simulink model "PMSLM_Close_Loop_MBDL4"  (R2026a)
settings: Solver=FixedStepDiscrete  StopTime=Inf  FixedStep=Ts  EnableMultiTasking=on
values from neighbouring files (symbols this model uses):
  ADC_GainA = 0.01664    [PMSLM_Init_Params_MBDL4.m]
  ADC_GainB = 0.01664    [PMSLM_Init_Params_MBDL4.m]
  ADC_GainC = 0.01664    [PMSLM_Init_Params_MBDL4.m]
  Close_Loop_EN = Simulink.Parameter    [PMSLM_Init_Params_MBDL4.m]
  CPU_Clock = 200e6    (= 200000000)    [PMSLM_Init_Params_MBDL4.m]    (also in init_PMLSM_ThreeLoop_Simple.m)
  delay_N = 50    [PMSLM_Init_Params_MBDL4.m]
  ENCON_Manual = Simulink.Parameter    [PMSLM_Init_Params_MBDL4.m]
  FReset_Manual = Simulink.Parameter    [PMSLM_Init_Params_MBDL4.m]
  GPIO30_PWM_OE_Disable = Simulink.Parameter    [PMSLM_Init_Params_MBDL4.m]
  Grating_Resolution_mm_per_count = 0.0001    [PMSLM_Init_Params_MBDL4.m]
  Hold_Ticks = 30000    [PMSLM_Init_Params_MBDL4.m]
  Id_Init_Step = Id_Init_Target / Ramp_Ticks    (= 5e-05)    [PMSLM_Init_Params_MBDL4.m]
  Id_Init_Target = 0.5    [PMSLM_Init_Params_MBDL4.m]
  Id_Ref_Set = Simulink.Parameter    [PMSLM_Init_Params_MBDL4.m]
  Init_Reset = Simulink.Parameter    [PMSLM_Init_Params_MBDL4.m]
  Init_Start = Simulink.Parameter    [PMSLM_Init_Params_MBDL4.m]
  Iq_fric_run = 0.05    [PMSLM_Init_Params_MBDL4.m]
  Iq_fric_start = 0.40    (= 0.4)    [PMSLM_Init_Params_MBDL4.m]
  Iq_int_limit = 0.10    (= 0.1)    [PMSLM_Init_Params_MBDL4.m]    (also in init_PMLSM_ThreeLoop_Simple.m = 0.5)
  Iq_Test_Mode = Simulink.Parameter    [PMSLM_Init_Params_MBDL4.m]
  Iq_Test_Ref = Simulink.Parameter    [PMSLM_Init_Params_MBDL4.m]
  Kaw_d = Kaw_q    (= 0.2)    [PMSLM_Init_Params_MBDL4.m]    (also in init_PMLSM_ThreeLoop_Simple.m = Tuning_Gains.Kaw_d)
  Kaw_q = 0.2    [PMSLM_Init_Params_MBDL4.m]    (also in init_PMLSM_ThreeLoop_Simple.m = Tuning_Gains.Kaw_q)
  Kaw_s = 0.4    [PMSLM_Init_Params_MBDL4.m]    (also in init_PMLSM_ThreeLoop_Simple.m = Tuning_Gains.Kaw_s)
  Ki_ACR = ACR_Commissioning_Scale*Ki_ACR_Baseline    (= 2962.5)    [PMSLM_Init_Params_MBDL4.m]    (also in init_PMLSM_ThreeLoop_Simple.m = Tuning_Gains.Ki_ACR; init_PMLSM_mil_test_params.m = Kp_ACR*PMLSM_Rs_ohm/PMLSM_Lq_H)
  Ki_ASR = 0.05    [PMSLM_Init_Params_MBDL4.m]    (also in init_PMLSM_ThreeLoop_Simple.m = Tuning_Gains.Ki_ASR)
  Kp_ACR = ACR_Commissioning_Scale*Kp_ACR_Baseline    (= 2.18125)    [PMSLM_Init_Params_MBDL4.m]    (also in init_PMLSM_ThreeLoop_Simple.m = Tuning_Gains.Kp_ACR; init_PMLSM_mil_test_params.m = PMLSM_Lq_H/(4*MIL_AUM3S4_Current_PI_xi^2*MIL_AUM3S4_Current_)
  Kp_ASR = 0.03    [PMSLM_Init_Params_MBDL4.m]    (also in init_PMLSM_ThreeLoop_Simple.m = Tuning_Gains.Kp_ASR)
  Kp_pos = 5    [PMSLM_Init_Params_MBDL4.m]    (also in init_PMLSM_ThreeLoop_Simple.m = Tuning_Gains.Kp_pos)
  OffsetCal_EN = Simulink.Parameter    [PMSLM_Init_Params_MBDL4.m]
  PI_Reset_EN = Simulink.Parameter    [PMSLM_Init_Params_MBDL4.m]
  PMLSM_Ld_H = Ld    (= 0.001745)    [PMSLM_Init_Params_MBDL4.m]    (also in init_PMLSM_ThreeLoop_Simple.m; init_PMLSM_plant_params.m)
  PMLSM_Lq_H = Lq    (= 0.001745)    [PMSLM_Init_Params_MBDL4.m]    (also in init_PMLSM_ThreeLoop_Simple.m; init_PMLSM_plant_params.m)
  PMLSM_psi_f_Wb = flux    (= 0.141)    [PMSLM_Init_Params_MBDL4.m]    (also in init_PMLSM_ThreeLoop_Simple.m; init_PMLSM_plant_params.m)
  Pos_deadband = 0.02    [PMSLM_Init_Params_MBDL4.m]    (also in init_PMLSM_ThreeLoop_Simple.m)
  Pos_Loop_EN = Simulink.Parameter    [PMSLM_Init_Params_MBDL4.m]
  qep_mid_cnt = 2147483648    [PMSLM_Init_Params_MBDL4.m]
  Ramp_Ticks = 10000    [PMSLM_Init_Params_MBDL4.m]
  RELCON_Manual = Simulink.Parameter    [PMSLM_Init_Params_MBDL4.m]
  Speed_loop_Iq_Limit = Iq_Limit    (= 0.3)    [PMSLM_Init_Params_MBDL4.m]    (also in init_PMLSM_ThreeLoop_Simple.m = 1)
  Tau_e_mm = 60    [PMSLM_Init_Params_MBDL4.m]
  theta_align_const = 0    [PMSLM_Init_Params_MBDL4.m]
  Theta_Offset_Fine = Simulink.Parameter    [PMSLM_Init_Params_MBDL4.m]
  Three_Current_Sampling_EN = Simulink.Parameter    [PMSLM_Init_Params_MBDL4.m]
  Ts = 1 / PWM_Freq    (= 0.0001)    [PMSLM_Init_Params_MBDL4.m]    (also in init_PMLSM_ThreeLoop_Simple.m)
  Ts_ACR = 1e-4    (= 0.0001)    [PMSLM_Init_Params_MBDL4.m]    (also in init_PMLSM_ThreeLoop_Simple.m)
  Ts_ASR = 1e-3    (= 0.001)    [PMSLM_Init_Params_MBDL4.m]    (also in init_PMLSM_ThreeLoop_Simple.m)
  Udc = 48    [PMSLM_Init_Params_MBDL4.m]    (also in init_PMLSM_ThreeLoop_Simple.m; init_PMLSM_mil_test_params.m)
  Uq_Zero_EN = 0：q 轴用正常 PI    [PMSLM_Init_Params_MBDL4.m]
  v_ff_eps = 0.5    [PMSLM_Init_Params_MBDL4.m]    (also in init_PMLSM_ThreeLoop_Simple.m)
  V_meas_max = 500    [PMSLM_Init_Params_MBDL4.m]
  v_meas_zero_eps = 0.5    [PMSLM_Init_Params_MBDL4.m]
  v_over_eps = 3    [PMSLM_Init_Params_MBDL4.m]    (also in init_PMLSM_ThreeLoop_Simple.m)
  V_pos_max_mmps = 10    [PMSLM_Init_Params_MBDL4.m]    (also in init_PMLSM_ThreeLoop_Simple.m = 20)
  v_ref_max = 20    [PMSLM_Init_Params_MBDL4.m]    (also in init_PMLSM_ThreeLoop_Simple.m)
  v_ref_set = Simulink.Parameter    [PMSLM_Init_Params_MBDL4.m]
  v_ref_set_step_dn = v_ref_set_rate_dn * Ts    (= 0.005)    [PMSLM_Init_Params_MBDL4.m]    (also in init_PMLSM_ThreeLoop_Simple.m)
  v_ref_set_step_up = v_ref_set_rate_up * Ts    (= 0.005)    [PMSLM_Init_Params_MBDL4.m]    (also in init_PMLSM_ThreeLoop_Simple.m)
  v_ref_zero_eps = 0.2    [PMSLM_Init_Params_MBDL4.m]    (also in init_PMLSM_ThreeLoop_Simple.m = 0)
  v_stick_off = 3.0    (= 3)    [PMSLM_Init_Params_MBDL4.m]
  v_stick_on = 1.0    (= 1)    [PMSLM_Init_Params_MBDL4.m]
  X_max_hard = 500    [PMSLM_Init_Params_MBDL4.m]
  X_max_soft = 470    [PMSLM_Init_Params_MBDL4.m]
  X_min_hard = -500    [PMSLM_Init_Params_MBDL4.m]
  X_min_soft = -470    [PMSLM_Init_Params_MBDL4.m]
  x_ref_mm = Simulink.Parameter    [PMSLM_Init_Params_MBDL4.m]
undefined symbols (not defined in the file or in its folder): bit, Down, GPTRIP1SEL, TZ1, Up
libraries: simulink x11, c2802xlib x6, c2838xlib x6, mcbeeMathTransformLib x2, c280xlib x1, mcbcontrolslib x1, svdschedulerlib x1
(part 2 of 2)

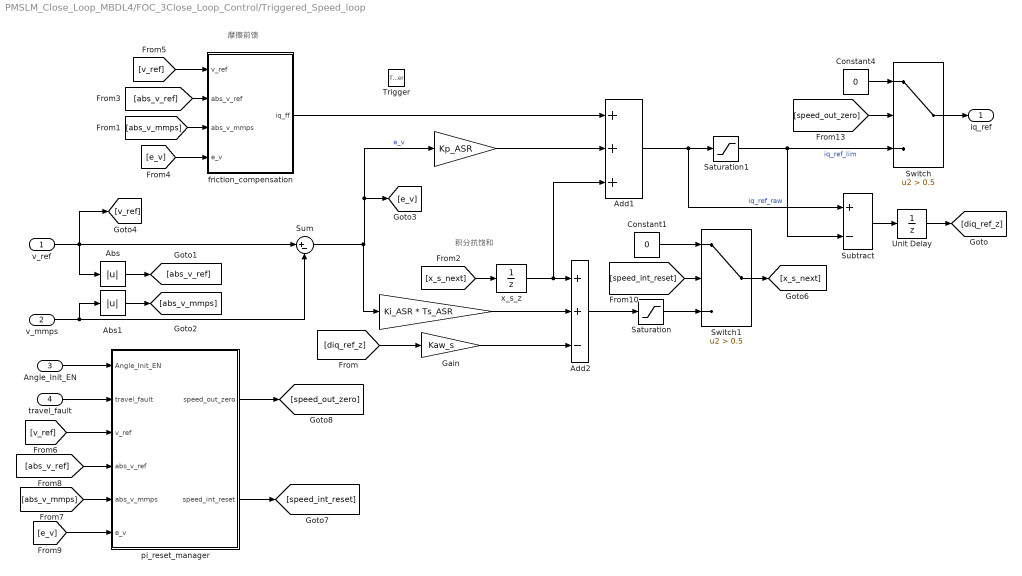
== system PMSLM_Close_Loop_MBDL4/FOC_3Close_Loop_Control/Triggered_Speed_loop ==
  note: 摩擦前馈
  note: 积分抗饱和
  v_ref : Inport
  v_mmps : Inport  Port=2
  Angle_Init_EN : Inport  Port=3
  travel_fault : Inport  Port=4
  Trigger : TriggerPort  VariantControl=(inherit)
  " " : Gain  Gain=Ki_ASR * Ts_ASR
  "  " : Gain  Gain=Kp_ASR
  Abs : Abs  SaturateOnIntegerOverflow=off
  Abs1 : Abs  SaturateOnIntegerOverflow=off
  Add1 : Sum  Inputs=+++
  Add2 : Sum  Inputs=++-
  Constant1 : Constant  Value=0
  Constant4 : Constant  Value=0
  Gain : Gain  Gain=Kaw_s
  Saturation : Saturate  UpperLimit=Iq_int_limit  LowerLimit=-Iq_int_limit
  Saturation1 : Saturate  UpperLimit=Speed_loop_Iq_Limit  LowerLimit=-Speed_loop_Iq_Limit
  Subtract : Sum  Inputs=+-
  Sum : Sum  Inputs=|+-
  Switch : Switch  Criteria=u2 > Threshold  Threshold=0.5  SaturateOnIntegerOverflow=off  InputSameDT=off
  Switch1 : Switch  Criteria=u2 > Threshold  Threshold=0.5  SaturateOnIntegerOverflow=off  InputSameDT=off
  Unit Delay : UnitDelay  SampleTime=-1
  friction_compensation : Subsystem
  pi_reset_manager : Subsystem
  x_s_z : UnitDelay  SampleTime=-1
  iq_ref : Outport
  wires:
  v_mmps/1 -> Sum/2, Abs1/1
  Sum/1 -> " "/1, [e_v], "  "/1  "e_v"
  Add1/1 -> Subtract/1, Saturation1/1  "iq_ref_raw"
  v_ref/1 -> [v_ref], Abs/1, Sum/1
  Saturation1/1 -> Subtract/2, Switch/3  "iq_ref_lim"
  [x_s_next] -> x_s_z/1
  Add2/1 -> Saturation/1
  Gain/1 -> Add2/3
  " "/1 -> Add2/2
  Subtract/1 -> Unit Delay/1
  Unit Delay/1 -> [diq_ref_z]
  [diq_ref_z] -> Gain/1
  Constant1/1 -> Switch1/1
  Switch/1 -> iq_ref/1
  Constant4/1 -> Switch/1
  "  "/1 -> Add1/2
  friction_compensation/1(iq_ff) -> Add1/1
  x_s_z/1 -> Add1/3, Add2/1
  [e_v] -> friction_compensation/4(e_v)
  [abs_v_mmps] -> friction_compensation/3(abs_v_mmps)
  [abs_v_ref] -> friction_compensation/2(abs_v_ref)
  Abs/1 -> [abs_v_ref]
  Abs1/1 -> [abs_v_mmps]
  Angle_Init_EN/1 -> pi_reset_manager/1(Angle_Init_EN)
  travel_fault/1 -> pi_reset_manager/2(travel_fault)
  [v_ref] -> friction_compensation/1(v_ref)
  [v_ref] -> pi_reset_manager/3(v_ref)
  [abs_v_mmps] -> pi_reset_manager/5(abs_v_mmps)
  [abs_v_ref] -> pi_reset_manager/4(abs_v_ref)
  [e_v] -> pi_reset_manager/6(e_v)
  [speed_out_zero] -> Switch/2
  pi_reset_manager/2(speed_int_reset) -> [speed_int_reset]
  pi_reset_manager/1(speed_out_zero) -> [speed_out_zero]
  [speed_int_reset] -> Switch1/2
  Switch1/1 -> [x_s_next]
  Saturation/1 -> Switch1/3

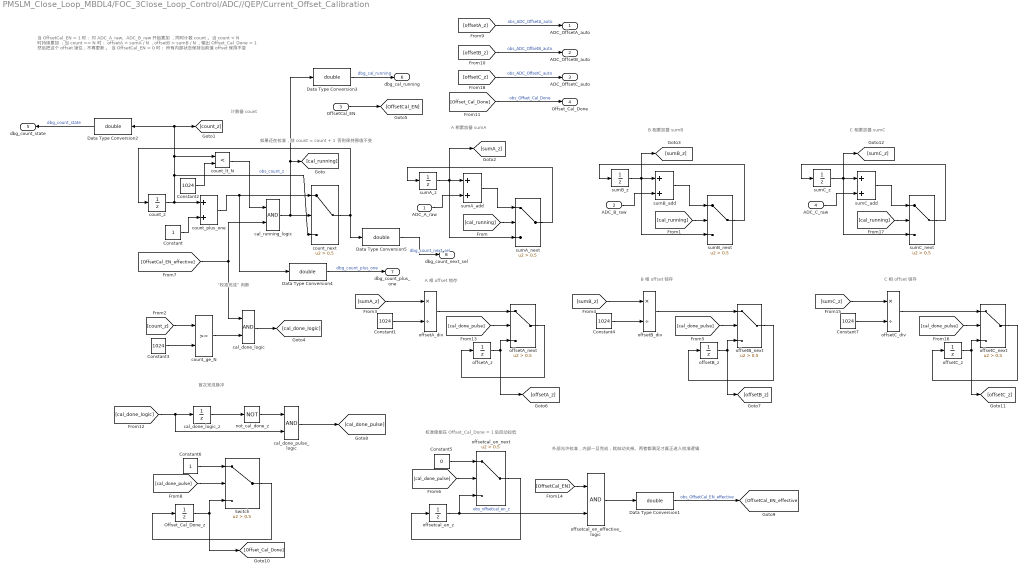
== system PMSLM_Close_Loop_MBDL4/FOC_3Close_Loop_Control/ADC//QEP/Current_Offset_Calibration ==
  note: 校准使能在 Offset_Cal_Done = 1 后自动拉低
  note: 外部允许校准，内部一旦完成，就自动关掉。两者都满足才真正进入校准逻辑
  note: 首次完成脉冲
  note: “校准完成” 判断
  note: B 相累加器 sumB
  note: A 相累加器 sumA
  note: 计数器 count
  note: B 相 offset 锁存
  note: A 相 offset 锁存
  note: 如果还在校准，就 count = count + 1 否则保持原值不变
  note: 当 OffsetCal_EN = 1 时：
      | 对 ADC_A_raw、ADC_B_raw 开始累加 ，同时计数 count 。当 count < N 时持续累加 ；当 count == N 时： offsetA = sumA / N ，offsetB = sumB / N ，输出 Offset_Cal_Done = 1 然后把这个 offset 锁住，不再更新 。
      |
      | 当 OffsetCal_EN = 0 时：
      | 所有内部状态保持当前值 offset 保持不变
  note: C 相 offset 锁存
  note: C 相累加器 sumC
  ADC_A_raw : Inport
  ADC_B_raw : Inport  Port=2
  OffsetCal_EN : Inport  Port=3
  ADC_C_raw : Inport  Port=4
  Constant : Constant  OutDataTypeStr=double
  Constant{1..4,7} (5 alike) : Constant  Value=1024  OutDataTypeStr=double
  Constant5 : Constant  Value=0  OutDataTypeStr=double
  Constant6 : Constant  OutDataTypeStr=double
  Data Type Conversion{1..5} (5 alike) : DataTypeConversion  OutDataTypeStr=double  SaturateOnIntegerOverflow=off  RndMeth=Floor
  Offset_Cal_Done_z : UnitDelay  SampleTime=-1
  Switch : Switch  Criteria=u2 > Threshold  Threshold=0.5  OutDataTypeStr=double  SaturateOnIntegerOverflow=off  InputSameDT=off
  cal_done_logic : Logic  AllPortsSameDT=off  OutDataTypeStr=boolean
  cal_done_logic_z : UnitDelay  SampleTime=-1
  cal_done_pulse_logic : Logic  AllPortsSameDT=off  OutDataTypeStr=boolean
  cal_running_logic : Logic  AllPortsSameDT=off  OutDataTypeStr=boolean
  count_ge_N : RelationalOperator  OutDataTypeStr=boolean  RndMeth=Simplest  InputSameDT=off
  count_lt_N : RelationalOperator  Operator=<  OutDataTypeStr=boolean  RndMeth=Simplest  InputSameDT=off
  count_next : Switch  Criteria=u2 > Threshold  Threshold=0.5  OutDataTypeStr=double  SaturateOnIntegerOverflow=off  InputSameDT=off
  count_plus_one : Sum
  count_z : UnitDelay  SampleTime=-1
  not_cal_done_z : Logic  Operator=NOT  AllPortsSameDT=off  OutDataTypeStr=boolean
  offsetA_div : Product  Inputs=*/
  offsetA_next : Switch  Criteria=u2 > Threshold  Threshold=0.5  OutDataTypeStr=double  SaturateOnIntegerOverflow=off  InputSameDT=off
  offsetA_z : UnitDelay  InitialCondition=2253  SampleTime=-1
  offsetB_div : Product  Inputs=*/
  offsetB_next : Switch  Criteria=u2 > Threshold  Threshold=0.5  OutDataTypeStr=double  SaturateOnIntegerOverflow=off  InputSameDT=off
  offsetB_z : UnitDelay  InitialCondition=2253  SampleTime=-1
  offsetC_div : Product  Inputs=*/
  offsetC_next : Switch  Criteria=u2 > Threshold  Threshold=0.5  OutDataTypeStr=double  SaturateOnIntegerOverflow=off  InputSameDT=off
  offsetC_z : UnitDelay  InitialCondition=2253  SampleTime=-1
  offsetcal_en_effective_logic : Logic  AllPortsSameDT=off  OutDataTypeStr=boolean
  offsetcal_en_next : Switch  Criteria=u2 > Threshold  Threshold=0.5  OutDataTypeStr=double  SaturateOnIntegerOverflow=off  InputSameDT=off
  offsetcal_en_z : UnitDelay  InitialCondition=1  SampleTime=-1
  sumA_add : Sum
  sumA_next : Switch  Criteria=u2 > Threshold  Threshold=0.5  OutDataTypeStr=double  SaturateOnIntegerOverflow=off  InputSameDT=off
  sumA_z : UnitDelay  SampleTime=-1
  sumB_add : Sum
  sumB_next : Switch  Criteria=u2 > Threshold  Threshold=0.5  OutDataTypeStr=double  SaturateOnIntegerOverflow=off  InputSameDT=off
  sumB_z : UnitDelay  SampleTime=-1
  sumC_add : Sum
  sumC_next : Switch  Criteria=u2 > Threshold  Threshold=0.5  OutDataTypeStr=double  SaturateOnIntegerOverflow=off  InputSameDT=off
  sumC_z : UnitDelay  SampleTime=-1
  ADC_OffsetA_auto : Outport
  ADC_OffsetB_auto : Outport  Port=2
  ADC_OffsetC_auto : Outport  Port=3
  Offset_Cal_Done : Outport  Port=4
  dbg_count_state : Outport  Port=5
  dbg_cal_running : Outport  Port=6
  dbg_count_plus_one : Outport  Port=7
  dbg_count_next_sel : Outport  Port=8
  wires:
  count_z/1 -> Data Type Conversion2/1, [count_z], count_lt_N/1, count_next/3, count_plus_one/1  "obs_count_z"
  Constant/1 -> count_plus_one/2
  Constant2/1 -> count_lt_N/2
  count_lt_N/1 -> cal_running_logic/1
  count_plus_one/1 -> Data Type Conversion4/1, count_next/1
  cal_running_logic/1 -> Data Type Conversion3/1, [cal_running], count_next/2
  count_next/1 -> count_z/1, Data Type Conversion5/1
  sumA_z/1 -> [sumA_z], sumA_next/3, sumA_add/1
  ADC_A_raw/1 -> sumA_add/2
  sumA_add/1 -> sumA_next/1
  [cal_running] -> sumA_next/2
  sumA_next/1 -> sumA_z/1
  sumB_next/1 -> sumB_z/1
  [cal_running] -> sumB_next/2
  sumB_add/1 -> sumB_next/1
  ADC_B_raw/1 -> sumB_add/2
  sumB_z/1 -> [sumB_z], sumB_next/3, sumB_add/1
  [count_z] -> count_ge_N/1
  Constant3/1 -> count_ge_N/2
  count_ge_N/1 -> cal_done_logic/2
  [sumA_z] -> offsetA_div/1
  Constant1/1 -> offsetA_div/2
  Constant4/1 -> offsetB_div/2
  [sumB_z] -> offsetB_div/1
  offsetA_div/1 -> offsetA_next/1
  cal_done_logic/1 -> [cal_done_logic]
  offsetA_z/1 -> [offsetA_z], offsetA_next/3
  offsetA_next/1 -> offsetA_z/1
  [cal_done_pulse] -> offsetB_next/2
  offsetB_z/1 -> [offsetB_z], offsetB_next/3
  offsetB_next/1 -> offsetB_z/1
  offsetB_div/1 -> offsetB_next/1
  OffsetCal_EN/1 -> [OffsetCal_EN]
  [offsetA_z] -> ADC_OffsetA_auto/1  "obs_ADC_OffsetA_auto"
  [offsetB_z] -> ADC_OffsetB_auto/1  "obs_ADC_OffsetB_auto"
  [cal_done_logic] -> cal_done_pulse_logic/2, cal_done_logic_z/1
  cal_done_logic_z/1 -> not_cal_done_z/1
  not_cal_done_z/1 -> cal_done_pulse_logic/1
  [cal_done_pulse] -> offsetA_next/2
  Constant5/1 -> offsetcal_en_next/1
  [cal_done_pulse] -> offsetcal_en_next/2
  offsetcal_en_z/1 -> offsetcal_en_effective_logic/2, offsetcal_en_next/3  "obs_offsetcal_en_z"
  offsetcal_en_next/1 -> offsetcal_en_z/1
  [OffsetCal_EN] -> offsetcal_en_effective_logic/1
  offsetcal_en_effective_logic/1 -> Data Type Conversion1/1
  [OffsetCal_EN_effective] -> cal_running_logic/2, cal_done_logic/1
  [Offset_Cal_Done] -> Offset_Cal_Done/1  "obs_Offset_Cal_Done"
  Data Type Conversion1/1 -> [OffsetCal_EN_effective]  "obs_OffsetCal_EN_effective"
  Data Type Conversion2/1 -> dbg_count_state/1  "dbg_count_state"
  Data Type Conversion3/1 -> dbg_cal_running/1  "dbg_cal_running"
  Data Type Conversion4/1 -> dbg_count_plus_one/1  "dbg_count_plus_one"
  Data Type Conversion5/1 -> dbg_count_next_sel/1  "dbg_count_next_sel"
  cal_done_pulse_logic/1 -> [cal_done_pulse]
  Constant6/1 -> Switch/1
  [cal_done_pulse] -> Switch/2
  Offset_Cal_Done_z/1 -> [Offset_Cal_Done], Switch/3
  Switch/1 -> Offset_Cal_Done_z/1
  offsetC_z/1 -> [offsetC_z], offsetC_next/3
  Constant7/1 -> offsetC_div/2
  [sumC_z] -> offsetC_div/1
  offsetC_div/1 -> offsetC_next/1
  offsetC_next/1 -> offsetC_z/1
  [cal_done_pulse] -> offsetC_next/2
  sumC_z/1 -> [sumC_z], sumC_next/3, sumC_add/1
  ADC_C_raw/1 -> sumC_add/2
  sumC_add/1 -> sumC_next/1
  sumC_next/1 -> sumC_z/1
  [cal_running] -> sumC_next/2
  [offsetC_z] -> ADC_OffsetC_auto/1  "obs_ADC_OffsetC_auto"

== system PMSLM_Close_Loop_MBDL4/FOC_3Close_Loop_Control/Caculate_measurement/IIR Filter ==
  In1 : Inport
  Reset : ResetPort  DisableCoverage=on
  IIR Filter : mcbcontrolslib/IIR Filter  VariantControl=Low Pass Filter  VariantSelect=Low-pass  FilterConstantInputType=Specify via dialog  Filter_constant=0.1  InitialOutput=Specify via dialog  InitialOutputValue=0  ExternalReset=none  advancedSettings=on  Ts=100e-6  cutOff_freq=176.8388
  Out1 : Outport
  wires:
  In1/1 -> IIR Filter/1
  IIR Filter/1 -> Out1/1

== system PMSLM_Close_Loop_MBDL4/FOC_3Close_Loop_Control/Controller_Driver_IO_Manager/External_Fault_Latch ==
  ERRI_raw : Inport  OutDataTypeStr=boolean  PortDimensions=1
  ERRU_raw : Inport  Port=2  OutDataTypeStr=boolean  PortDimensions=1
  ERRI_Active_Low : Logic  Operator=NOT  IconShape=distinctive
  ERRU_Active_Low : Logic  Operator=NOT  IconShape=distinctive
  External_Fault_Latch_OR : Logic  Operator=OR  IconShape=distinctive
  External_Fault_Latch_Z : UnitDelay  InitialCondition=false  SampleTime=-1
  External_Fault_OR : Logic  Operator=OR  IconShape=distinctive
  external_fault_latch : Outport  OutDataTypeStr=boolean  PortDimensions=1
  wires:
  External_Fault_Latch_OR/1 -> External_Fault_Latch_Z/1, external_fault_latch/1
  External_Fault_Latch_Z/1 -> External_Fault_Latch_OR/2
  External_Fault_OR/1 -> External_Fault_Latch_OR/1
  ERRU_Active_Low/1 -> External_Fault_OR/2
  ERRI_Active_Low/1 -> External_Fault_OR/1
  ERRU_raw/1 -> ERRU_Active_Low/1
  ERRI_raw/1 -> ERRI_Active_Low/1

== system PMSLM_Close_Loop_MBDL4/FOC_3Close_Loop_Control/FOC_Algorithm/Clack ==
  note: alpha=(A-0.5*(B+C))*2/3
      | Beta=sqrt(3)/2*(B-C)*2/3
  ia : Inport
  ib : Inport  Port=2
  ic : Inport  Port=3
  Add : Sum  Inputs=+--
  Add1 : Sum  Inputs=+-
  Gain : Gain  Gain=0.5
  Gain1 : Gain  Gain=0.5
  Gain2 : Gain  Gain=2/3
  Gain3 : Gain  Gain=1/sqrt(3)
  ialpha : Outport
  ibeta : Outport  Port=2
  wires:
  Gain1/1 -> Add/3
  ia/1 -> Add/1
  ib/1 -> Add1/1, Gain/1
  Add1/1 -> Gain3/1
  ic/1 -> Add1/2, Gain1/1
  Gain3/1 -> ibeta/1  "ibeta"
  Add/1 -> Gain2/1
  Gain2/1 -> ialpha/1  "ialf"
  Gain/1 -> Add/2

== system PMSLM_Close_Loop_MBDL4/FOC_3Close_Loop_Control/FOC_Algorithm/SVPWMG ==
  Valpha : Inport
  Vbeta : Inport  Port=2
  Duty Calculate : Subsystem  TreatAsAtomicUnit=on  RTWFcnName=Duty_Caculate_Fun
      settings: RTWFcnNameOpts=User specified
  Sector Caculate : Subsystem  TreatAsAtomicUnit=on  RTWFcnName=Sector_Caculate_Fun
      settings: RTWFcnNameOpts=User specified
  T1T2 Calculate : Subsystem  TreatAsAtomicUnit=on  RTWFcnName=T1T2Caculate_Fun
      settings: RTWFcnNameOpts=User specified
  Udc : Constant  Value=Udc
  XYZ Calculate : Subsystem  TreatAsAtomicUnit=on  RTWFcnName=XYZ_Caculate_Fun
      settings: RTWFcnNameOpts=User specified
  Duty_A : Outport
  Duty_B : Outport  Port=2
  Duty_C : Outport  Port=3
  "N " : Outport  Port=4
  wires:
  Vbeta/1 -> Sector Caculate/2(Ubeta), XYZ Calculate/2(Ubeta)
  T1T2 Calculate/1(T1) -> Duty Calculate/2(T1)
  Valpha/1 -> Sector Caculate/1(Ualpha), XYZ Calculate/1(Ualpha)
  T1T2 Calculate/2(T2) -> Duty Calculate/3(T2)
  Sector Caculate/1("N ") -> "N "/1, Duty Calculate/1(N), T1T2 Calculate/1(N)
  Udc/1 -> XYZ Calculate/3(Udc)
  XYZ Calculate/1(X) -> T1T2 Calculate/2(X)
  XYZ Calculate/2(Y) -> T1T2 Calculate/3(Y)
  XYZ Calculate/3(Z) -> T1T2 Calculate/4(Z)
  Duty Calculate/1(Duty_U) -> Duty_A/1
  Duty Calculate/2(Duty_V) -> Duty_B/1
  Duty Calculate/3(Duty_W) -> Duty_C/1

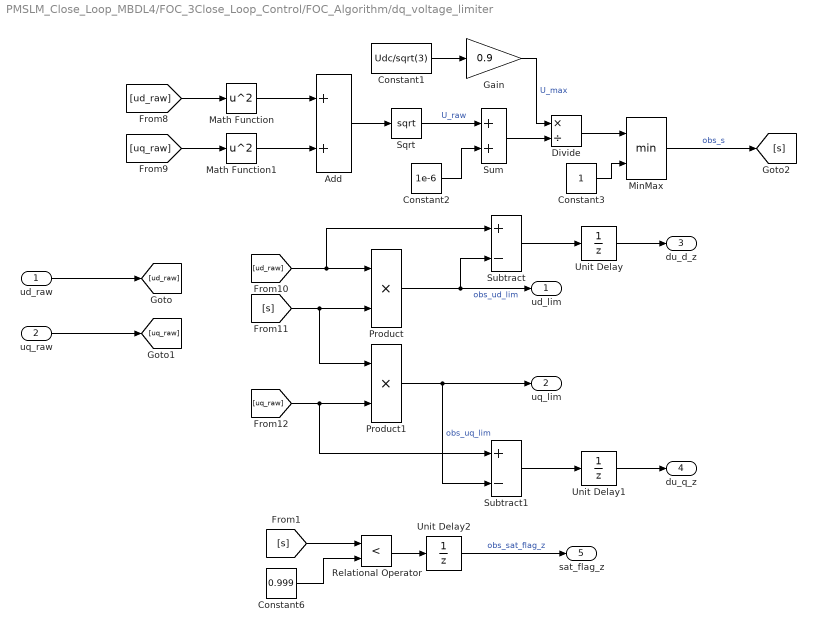
== system PMSLM_Close_Loop_MBDL4/FOC_3Close_Loop_Control/FOC_Algorithm/dq_voltage_limiter ==
  ud_raw : Inport
  uq_raw : Inport  Port=2
  Add : Sum
  Constant1 : Constant  Value=Udc/sqrt(3)  OutDataTypeStr=double
  Constant2 : Constant  Value=1e-6  OutDataTypeStr=double
  Constant3 : Constant  OutDataTypeStr=double
  Constant6 : Constant  Value=0.999
  Divide : Product  Inputs=*/  OutDataTypeStr=double
  Gain : Gain  Gain=0.9  OutDataTypeStr=double
  Math Function : Math  Operator=square
  Math Function1 : Math  Operator=square
  MinMax : MinMax  Inputs=2
  Product : Product
  Product1 : Product  OutDataTypeStr=double
  Relational Operator : RelationalOperator  Operator=<  OutDataTypeStr=boolean  RndMeth=Simplest  InputSameDT=off
  Sqrt : Sqrt
  Subtract : Sum  Inputs=+-
  Subtract1 : Sum  Inputs=+-
  Sum : Sum
  Unit Delay : UnitDelay  SampleTime=-1
  Unit Delay1 : UnitDelay  SampleTime=-1
  Unit Delay2 : UnitDelay  SampleTime=-1
  ud_lim : Outport
  uq_lim : Outport  Port=2
  du_d_z : Outport  Port=3
  du_q_z : Outport  Port=4
  sat_flag_z : Outport  Port=5
  wires:
  Sum/1 -> Divide/2
  Constant2/1 -> Sum/2
  Constant3/1 -> MinMax/2
  Add/1 -> Sqrt/1
  Constant1/1 -> Gain/1
  Divide/1 -> MinMax/1
  Gain/1 -> Divide/1  "U_max"
  Sqrt/1 -> Sum/1  "U_raw"
  Math Function1/1 -> Add/2
  Math Function/1 -> Add/1
  [uq_raw] -> Math Function1/1
  [ud_raw] -> Math Function/1
  MinMax/1 -> [s]  "obs_s"
  Product1/1 -> uq_lim/1, Subtract1/2  "obs_uq_lim"
  [s] -> Product1/1, Product/2
  [ud_raw] -> Subtract/1, Product/1
  Product/1 -> Subtract/2, ud_lim/1  "obs_ud_lim"
  [uq_raw] -> Subtract1/1, Product1/2
  Subtract/1 -> Unit Delay/1
  Subtract1/1 -> Unit Delay1/1
  ud_raw/1 -> [ud_raw]
  uq_raw/1 -> [uq_raw]
  Unit Delay/1 -> du_d_z/1
  Unit Delay1/1 -> du_q_z/1
  Constant6/1 -> Relational Operator/2
  [s] -> Relational Operator/1
  Relational Operator/1 -> Unit Delay2/1
  Unit Delay2/1 -> sat_flag_z/1  "obs_sat_flag_z"

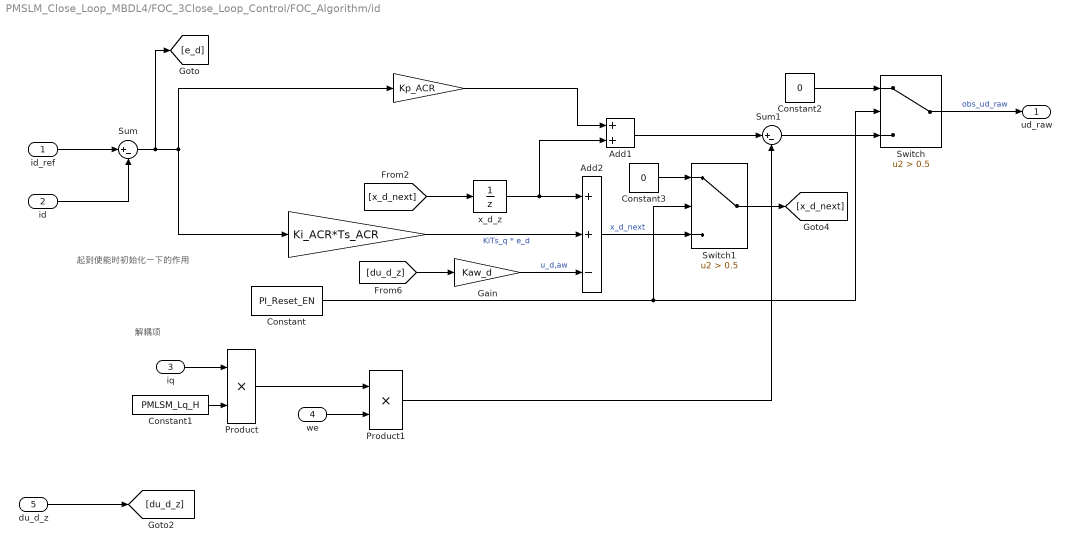
== system PMSLM_Close_Loop_MBDL4/FOC_3Close_Loop_Control/FOC_Algorithm/id ==
  note: 解耦项
  note: 起到使能时初始化一下的作用
  id_ref : Inport
  id : Inport  Port=2
  iq : Inport  Port=3
  we : Inport  Port=4
  du_d_z : Inport  Port=5
  " " : Gain  Gain=Ki_ACR*Ts_ACR
  "  " : Gain  Gain=Kp_ACR
  Add1 : Sum
  Add2 : Sum  Inputs=++-
  Constant : Constant  Value=PI_Reset_EN
  Constant1 : Constant  Value=PMLSM_Lq_H
  Constant2 : Constant  Value=0
  Constant3 : Constant  Value=0
  Gain : Gain  Gain=Kaw_d
  Product : Product
  Product1 : Product
  Sum : Sum  Inputs=|+-
  Sum1 : Sum  Inputs=|+-
  Switch : Switch  Criteria=u2 > Threshold  Threshold=0.5  SaturateOnIntegerOverflow=off  InputSameDT=off
  Switch1 : Switch  Criteria=u2 > Threshold  Threshold=0.5  SaturateOnIntegerOverflow=off  InputSameDT=off
  x_d_z : UnitDelay  SampleTime=-1
  ud_raw : Outport
  wires:
  iq/1 -> Product/1
  id_ref/1 -> Sum/1
  id/1 -> Sum/2
  Sum/1 -> [e_d], " "/1, "  "/1
  Product1/1 -> Sum1/2
  we/1 -> Product1/2
  Product/1 -> Product1/1
  Add1/1 -> Sum1/1
  Constant1/1 -> Product/2
  Constant/1 -> Switch1/2, Switch/2
  "  "/1 -> Add1/1
  Constant2/1 -> Switch/1
  Sum1/1 -> Switch/3
  Switch/1 -> ud_raw/1  "obs_ud_raw"
  du_d_z/1 -> [du_d_z]
  x_d_z/1 -> Add1/2, Add2/1
  [x_d_next] -> x_d_z/1
  Add2/1 -> Switch1/3  "x_d_next"
  Gain/1 -> Add2/3  "u_d,aw"
  [du_d_z] -> Gain/1
  " "/1 -> Add2/2  "KiTs_q * e_d"
  Constant3/1 -> Switch1/1
  Switch1/1 -> [x_d_next]

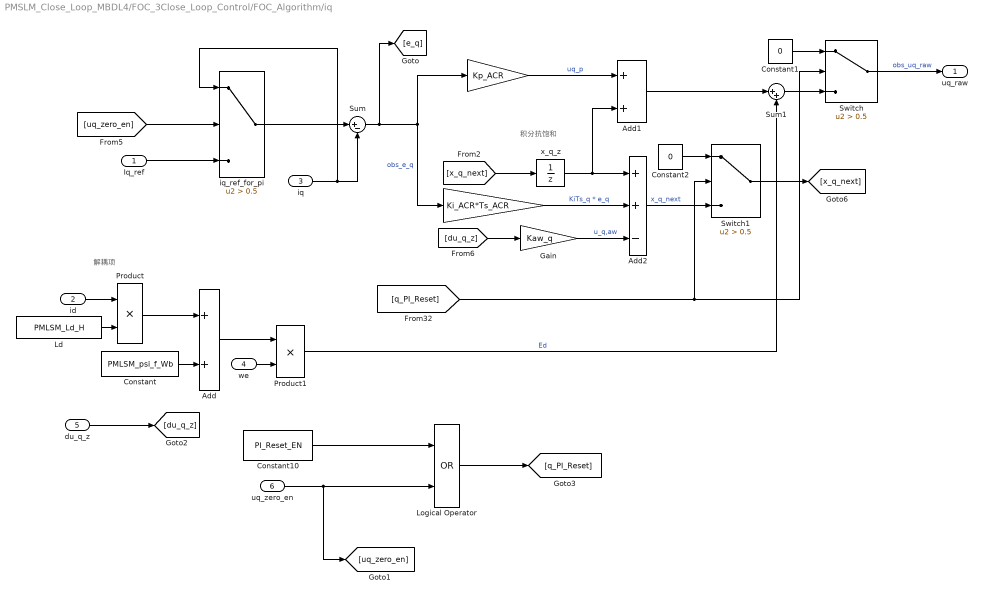
== system PMSLM_Close_Loop_MBDL4/FOC_3Close_Loop_Control/FOC_Algorithm/iq ==
  note: 解耦项
  note: 积分抗饱和
  Iq_ref : Inport
  id : Inport  Port=2
  iq : Inport  Port=3
  we : Inport  Port=4
  du_q_z : Inport  Port=5
  uq_zero_en : Inport  Port=6
  " " : Gain  Gain=Ki_ACR*Ts_ACR
  "  " : Gain  Gain=Kp_ACR
  Add : Sum
  Add1 : Sum
  Add2 : Sum  Inputs=++-
  Constant : Constant  Value=PMLSM_psi_f_Wb
  Constant1 : Constant  Value=0
  Constant10 : Constant  Value=PI_Reset_EN
  Constant2 : Constant  Value=0
  Gain : Gain  Gain=Kaw_q
  Ld : Constant  Value=PMLSM_Ld_H
  Logical Operator : Logic  Operator=OR  AllPortsSameDT=off  OutDataTypeStr=boolean
  Product : Product
  Product1 : Product
  Sum : Sum  Inputs=|+-
  Sum1 : Sum  Inputs=|++
  Switch : Switch  Criteria=u2 > Threshold  Threshold=0.5  SaturateOnIntegerOverflow=off  InputSameDT=off
  Switch1 : Switch  Criteria=u2 > Threshold  Threshold=0.5  SaturateOnIntegerOverflow=off  InputSameDT=off
  iq_ref_for_pi : Switch  Criteria=u2 > Threshold  Threshold=0.5  SaturateOnIntegerOverflow=off  InputSameDT=off
  x_q_z : UnitDelay  SampleTime=-1
  uq_raw : Outport
  wires:
  Product1/1 -> Sum1/2  "Ed"
  we/1 -> Product1/2
  Add1/1 -> Sum1/1
  iq/1 -> iq_ref_for_pi/1, Sum/2
  id/1 -> Product/1
  Ld/1 -> Product/2
  Product/1 -> Add/1
  Constant/1 -> Add/2
  Add/1 -> Product1/1
  Sum/1 -> [e_q], "  "/1, " "/1  "obs_e_q"
  "  "/1 -> Add1/1  "uq_p"
  Constant1/1 -> Switch/1
  Switch/1 -> uq_raw/1  "obs_uq_raw"
  Sum1/1 -> Switch/3
  [q_PI_Reset] -> Switch/2, Switch1/2
  du_q_z/1 -> [du_q_z]
  [uq_zero_en] -> iq_ref_for_pi/2
  Iq_ref/1 -> iq_ref_for_pi/3
  iq_ref_for_pi/1 -> Sum/1
  [du_q_z] -> Gain/1
  Gain/1 -> Add2/3  "u_q,aw"
  " "/1 -> Add2/2  "KiTs_q * e_q"
  x_q_z/1 -> Add1/2, Add2/1
  Constant2/1 -> Switch1/1
  Add2/1 -> Switch1/3  "x_q_next"
  Switch1/1 -> [x_q_next]
  [x_q_next] -> x_q_z/1
  uq_zero_en/1 -> [uq_zero_en], Logical Operator/2
  Constant10/1 -> Logical Operator/1
  Logical Operator/1 -> [q_PI_Reset]

== system PMSLM_Close_Loop_MBDL4/FOC_3Close_Loop_Control/Reference_Manager/v_ref_set_slew_limiter ==
  v_ref_set : Inport
  Add : Sum
  Saturation : Saturate  UpperLimit=v_ref_set_step_up  LowerLimit=-v_ref_set_step_dn
  Subtract : Sum  Inputs=+-
  v_ref_set_lim_z : UnitDelay  SampleTime=-1
  v_ref_set_limited : Outport
  wires:
  v_ref_set_lim_z/1 -> Add/2, Subtract/2
  v_ref_set/1 -> Subtract/1
  Saturation/1 -> Add/1
  Subtract/1 -> Saturation/1
  Add/1 -> v_ref_set_limited/1, v_ref_set_lim_z/1

== system PMSLM_Close_Loop_MBDL4/FOC_3Close_Loop_Control/Triggered_Speed_loop/friction_compensation ==
  note: if start_mode == 1
      | 	iq_fric_mag = Iq_fric_start;
      | else
      | 	iq_fric_mag = Iq_fric_run;
      |
      | if ff_enable
      | 	iq_ff = iq_fric_mag * sign(v_ref);
      |  else
      | 	iq_ff = 0;
  v_ref : Inport
  abs_v_ref : Inport  Port=2
  abs_v_mmps : Inport  Port=3
  e_v : Inport  Port=4
  Compare To Constant1 : simulink/Logic and Bit Operations/Compare To Constant  relop=>  const=-v_over_eps  OutDataTypeStr=boolean
  Compare To Constant2 : simulink/Logic and Bit Operations/Compare To Constant  relop=>  const=v_ff_eps  OutDataTypeStr=boolean
  Constant1 : Constant  Value=Iq_fric_start
  Constant5 : Constant  Value=0
  Constant6 : Constant  Value=Iq_fric_run
  Gain : Gain  Gain=-1
  Logical Operator : Logic  AllPortsSameDT=off  OutDataTypeStr=boolean
  Product : Product
  Product1 : Product
  Product2 : Product
  Relay : Relay  OnSwitchValue=-v_stick_on  OffSwitchValue=-v_stick_off
  Sign : Signum
  Sign1 : Signum
  Switch : Switch  Criteria=u2 > Threshold  Threshold=0.5  SaturateOnIntegerOverflow=off  InputSameDT=off
  Switch2 : Switch  Criteria=u2 > Threshold  Threshold=0.5  SaturateOnIntegerOverflow=off  InputSameDT=off
  iq_ff : Outport
  wires:
  v_ref/1 -> Sign/1, Sign1/1
  Sign/1 -> Product2/1, Product/1
  Constant5/1 -> Switch2/3
  Constant6/1 -> Product/2
  abs_v_ref/1 -> Compare To Constant2/1
  Switch2/1 -> iq_ff/1  "iq_ff"
  Switch/1 -> Switch2/1
  Product/1 -> Switch/3
  Sign1/1 -> Product1/1
  Constant1/1 -> Product1/2
  Product1/1 -> Switch/1
  e_v/1 -> Product2/2
  Product2/1 -> Compare To Constant1/1
  Compare To Constant2/1 -> Logical Operator/1
  Compare To Constant1/1 -> Logical Operator/2
  Logical Operator/1 -> Switch2/2  "ff_enable"
  abs_v_mmps/1 -> Gain/1
  Relay/1 -> Switch/2  "fric_start_mode"
  Gain/1 -> Relay/1

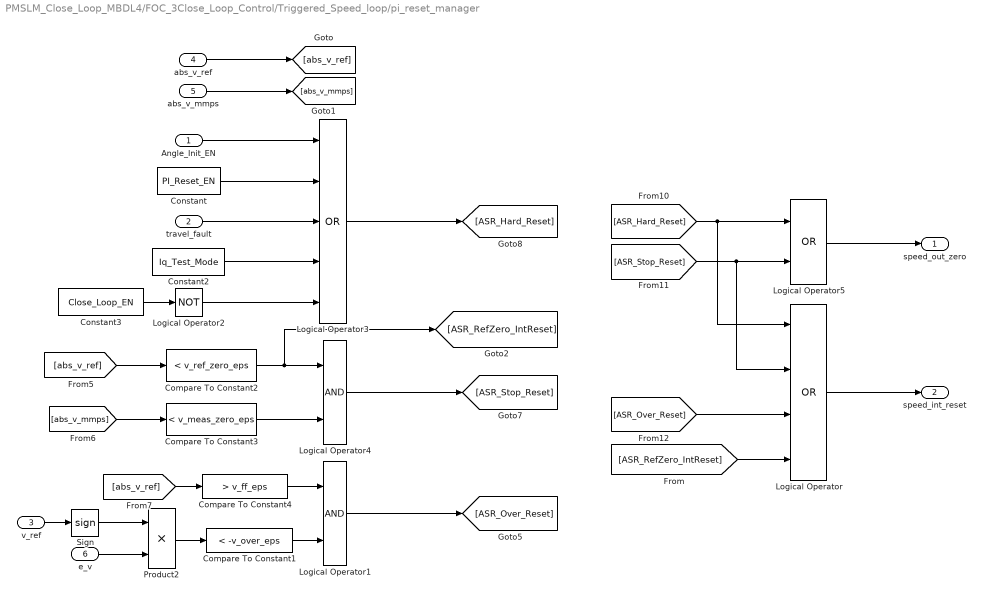
== system PMSLM_Close_Loop_MBDL4/FOC_3Close_Loop_Control/Triggered_Speed_loop/pi_reset_manager ==
  Angle_Init_EN : Inport
  travel_fault : Inport  Port=2
  v_ref : Inport  Port=3
  abs_v_ref : Inport  Port=4
  abs_v_mmps : Inport  Port=5
  e_v : Inport  Port=6
  Compare To Constant1 : simulink/Logic and Bit Operations/Compare To Constant  relop=<  const=-v_over_eps  OutDataTypeStr=boolean
  Compare To Constant2 : simulink/Logic and Bit Operations/Compare To Constant  relop=<  const=v_ref_zero_eps  OutDataTypeStr=boolean
  Compare To Constant3 : simulink/Logic and Bit Operations/Compare To Constant  relop=<  const=v_meas_zero_eps  OutDataTypeStr=boolean
  Compare To Constant4 : simulink/Logic and Bit Operations/Compare To Constant  relop=>  const=v_ff_eps  OutDataTypeStr=boolean
  Constant : Constant  Value=PI_Reset_EN
  Constant2 : Constant  Value=Iq_Test_Mode
  Constant3 : Constant  Value=Close_Loop_EN
  Logical Operator : Logic  Operator=OR  Inputs=4  AllPortsSameDT=off  OutDataTypeStr=boolean
  Logical Operator1 : Logic  AllPortsSameDT=off  OutDataTypeStr=boolean
  Logical Operator2 : Logic  Operator=NOT  AllPortsSameDT=off  OutDataTypeStr=boolean
  Logical Operator3 : Logic  Operator=OR  Inputs=5  AllPortsSameDT=off  OutDataTypeStr=boolean
  Logical Operator4 : Logic  AllPortsSameDT=off  OutDataTypeStr=boolean
  Logical Operator5 : Logic  Operator=OR  AllPortsSameDT=off  OutDataTypeStr=boolean
  Product2 : Product
  Sign : Signum
  speed_out_zero : Outport
  speed_int_reset : Outport  Port=2
  wires:
  Compare To Constant2/1 -> [ASR_RefZero_IntReset], Logical Operator4/1
  [abs_v_ref] -> Compare To Constant2/1
  Logical Operator2/1 -> Logical Operator3/5
  [abs_v_mmps] -> Compare To Constant3/1
  [abs_v_ref] -> Compare To Constant4/1
  e_v/1 -> Product2/2
  travel_fault/1 -> Logical Operator3/3
  Constant2/1 -> Logical Operator3/4
  Constant3/1 -> Logical Operator2/1
  Sign/1 -> Product2/1
  Constant/1 -> Logical Operator3/2
  Product2/1 -> Compare To Constant1/1
  Compare To Constant1/1 -> Logical Operator1/2
  Compare To Constant4/1 -> Logical Operator1/1
  Angle_Init_EN/1 -> Logical Operator3/1
  v_ref/1 -> Sign/1
  abs_v_ref/1 -> [abs_v_ref]
  abs_v_mmps/1 -> [abs_v_mmps]
  Compare To Constant3/1 -> Logical Operator4/2
  Logical Operator3/1 -> [ASR_Hard_Reset]
  Logical Operator5/1 -> speed_out_zero/1
  Logical Operator4/1 -> [ASR_Stop_Reset]
  [ASR_Stop_Reset] -> Logical Operator5/2, Logical Operator/2
  [ASR_Hard_Reset] -> Logical Operator5/1, Logical Operator/1
  [ASR_Over_Reset] -> Logical Operator/3
  Logical Operator/1 -> speed_int_reset/1
  Logical Operator1/1 -> [ASR_Over_Reset]
  [ASR_RefZero_IntReset] -> Logical Operator/4

== system PMSLM_Close_Loop_MBDL4/FOC_3Close_Loop_Control/FOC_Algorithm/SVPWMG/Duty Calculate ==
  N : Inport
  T1 : Inport  Port=2
  T2 : Inport  Port=3
  Constant : Constant  Value=Ts
  Fcn : Fcn  Expr=(u[3]-u[1]-u[2])/4
  Fcn1 : Fcn  Expr=(u[3]+u[1]-u[2])/4
  Fcn2 : Fcn  Expr=(u[3]+u[2]+u[1])/4
  Gain : Gain  Gain=CPU_Clock
  Gain1 : Gain  Gain=CPU_Clock
  Gain2 : Gain  Gain=CPU_Clock
  Multiport Switch : MultiPortSwitch  Inputs=6  SaturateOnIntegerOverflow=off  InputSameDT=off
  Multiport Switch1 : MultiPortSwitch  Inputs=6  SaturateOnIntegerOverflow=off  InputSameDT=off
  Multiport Switch2 : MultiPortSwitch  Inputs=6  SaturateOnIntegerOverflow=off  InputSameDT=off
  Mux : Mux  Inputs=3
  Duty_U : Outport
  Duty_V : Outport  Port=2
  Duty_W : Outport  Port=3
  wires:
  Mux/1 -> Fcn2/1, Fcn/1, Fcn1/1
  Constant/1 -> Mux/3
  T2/1 -> Mux/2
  T1/1 -> Mux/1
  Multiport Switch2/1 -> Gain2/1
  Multiport Switch1/1 -> Gain1/1
  Multiport Switch/1 -> Gain/1
  Fcn/1 -> Multiport Switch/3, Multiport Switch/4, Multiport Switch1/6, Multiport Switch2/5, Multiport Switch2/7, Multiport Switch1/2
  Fcn1/1 -> Multiport Switch1/5, Multiport Switch2/3, Multiport Switch2/6, Multiport Switch1/4, Multiport Switch/7, Multiport Switch/2
  Fcn2/1 -> Multiport Switch/5, Multiport Switch/6, Multiport Switch1/3, Multiport Switch1/7, Multiport Switch2/2, Multiport Switch2/4
  N/1 -> Multiport Switch2/1, Multiport Switch1/1, Multiport Switch/1
  Gain/1 -> Duty_U/1  "DutyU"
  Gain1/1 -> Duty_V/1  "DutyV"
  Gain2/1 -> Duty_W/1  "DutyW"

== system PMSLM_Close_Loop_MBDL4/FOC_3Close_Loop_Control/FOC_Algorithm/SVPWMG/Sector Caculate ==
  Ualpha : Inport
  Ubeta : Inport  Port=2
  B0 : Fcn  Expr=u[2]
  B1 : Fcn  Expr=u[1]*0.866-0.5*u[2]
  B2 : Fcn  Expr=-u[1]*0.866-u[2]*0.5
  Constant : Constant
  Constant1 : Constant  Value=0
  Mux : Mux  Inputs=2
  Mux1 : Mux  Inputs=3
  N : Fcn  Expr=4*u[3]+2*u[2]+u[1]
  Switch : Switch  Criteria=u2 > Threshold  SaturateOnIntegerOverflow=off  InputSameDT=off
  Switch1 : Switch  SaturateOnIntegerOverflow=off  InputSameDT=off
  Switch2 : Switch  Criteria=u2 > Threshold  SaturateOnIntegerOverflow=off  InputSameDT=off
  "N " : Outport  VectorParamsAs1DForOutWhenUnconnected=off
  wires:
  Switch2/1 -> Mux1/3
  Switch/1 -> Mux1/1
  Ualpha/1 -> Mux/1
  Ubeta/1 -> Mux/2
  Mux/1 -> B2/1, B1/1, B0/1
  B0/1 -> Switch/2
  B1/1 -> Switch1/2
  B2/1 -> Switch2/2
  Constant/1 -> Switch/1, Switch2/1, Switch1/1
  Constant1/1 -> Switch/3, Switch1/3, Switch2/3
  Switch1/1 -> Mux1/2
  Mux1/1 -> N/1
  N/1 -> "N "/1  "N"

== system PMSLM_Close_Loop_MBDL4/FOC_3Close_Loop_Control/FOC_Algorithm/SVPWMG/T1T2 Calculate ==
  N : Inport
  X : Inport  Port=2
  Y : Inport  Port=3
  Z : Inport  Port=4
  Constant : Constant  Value=Ts
  Fcn : Fcn  Expr=u(3)-u(2)-u(1)
  Fcn1 : Fcn  Expr=u(1)*u(3)/(u(1)+u(2))
  Fcn2 : Fcn  Expr=u(2)*u(3)/(u(1)+u(2))
  Gain : Gain  Gain=-1
  Gain1 : Gain  Gain=-1
  Gain2 : Gain  Gain=-1
  Multiport Switch : MultiPortSwitch  Inputs=6  SaturateOnIntegerOverflow=off  InputSameDT=off
  Multiport Switch1 : MultiPortSwitch  Inputs=6  SaturateOnIntegerOverflow=off  InputSameDT=off
  Mux : Mux  Inputs=3
  Switch : Switch  SaturateOnIntegerOverflow=off  InputSameDT=off
  Switch1 : Switch  Criteria=u2 > Threshold  SaturateOnIntegerOverflow=off  InputSameDT=off
  T1 : Outport  VectorParamsAs1DForOutWhenUnconnected=off
  T2 : Outport  Port=2  VectorParamsAs1DForOutWhenUnconnected=off
  wires:
  Constant/1 -> Mux/3
  Switch1/1 -> T2/1  "T2"
  Switch/1 -> T1/1  "T1"
  Fcn2/1 -> Switch1/3
  Fcn1/1 -> Switch/3
  Fcn/1 -> Switch/2, Switch1/2
  Mux/1 -> Fcn1/1, Fcn/1, Fcn2/1
  Multiport Switch/1 -> Switch/1, Mux/1
  Multiport Switch1/1 -> Switch1/1, Mux/2
  N/1 -> Multiport Switch/1, Multiport Switch1/1
  Y/1 -> Multiport Switch/3, Multiport Switch1/2, Gain1/1
  Z/1 -> Multiport Switch1/5, Multiport Switch/2, Gain2/1
  X/1 -> Gain/1, Multiport Switch/6, Multiport Switch1/4
  Gain/1 -> Multiport Switch1/3, Multiport Switch/5
  Gain2/1 -> Multiport Switch/4, Multiport Switch1/7
  Gain1/1 -> Multiport Switch1/6, Multiport Switch/7

== system PMSLM_Close_Loop_MBDL4/FOC_3Close_Loop_Control/FOC_Algorithm/SVPWMG/XYZ Calculate ==
  Ualpha : Inport
  Ubeta : Inport  Port=2
  Udc : Inport  Port=3
  Add : Sum
  Add1 : Sum  Inputs=+-
  Constant1 : Constant  Value=Ts
  Gain : Gain  Gain=3/2
  Gain1 : Gain  Gain=1.7321
  Gain2 : Gain  Gain=0.866
  Math Function : Math  Operator=reciprocal
  Product{,1..3} (4 alike) : Product
  X : Outport
  Y : Outport  Port=2
  Z : Outport  Port=3
  wires:
  Ualpha/1 -> Gain/1
  Udc/1 -> Math Function/1
  Math Function/1 -> Product/2
  Ubeta/1 -> Gain2/1, Gain1/1
  Gain1/1 -> Product1/1
  Product/1 -> Product2/2, Product3/2, Product1/2
  Gain2/1 -> Add/1, Add1/1
  Gain/1 -> Add1/2, Add/2
  Product1/1 -> X/1  "X"
  Add/1 -> Product3/1
  Add1/1 -> Product2/1
  Product2/1 -> Z/1  "Z"
  Product3/1 -> Y/1  "Y"
  Constant1/1 -> Product/1

== matlab function PMSLM_Close_Loop_MBDL4/FOC_3Close_Loop_Control/Travel_Safety_Manager ==
  data: v_ref_safe output; x_mm input; travel_fault_latch output; v_ref input; X_max_soft input; X_min_soft input; X_max_hard input; X_min_hard input; travel_fault_latch_z input
function [v_ref_safe, travel_fault_latch] = Travel_Safety_Manager( ...
    x_mm, v_ref, X_max_soft, X_min_soft, X_max_hard, X_min_hard, travel_fault_latch_z)
% PMLSM travel safety manager
% 功能：
% 1. 软限位：只限制继续向越界方向运动，不触发硬关断
% 2. 硬限位：触发 travel_fault_latch，锁存故障
% 3. travel_fault_latch = 1 后，v_ref_safe 强制为 0
% 注意：
% 当前版本没有 fault_reset 输入，硬限位故障一旦触发，
% 只能通过 DSP 复位/重新运行程序清除。
% 速度方向判断死区，单位 mm/s
V_eps = 1.0;

% ---------- 1. 硬限位检测 ----------
hard_hi = (x_mm >= X_max_hard);
hard_lo = (x_mm <= X_min_hard);
hard_fault_raw = hard_hi || hard_lo;

% ---------- 2. 外部锁存 ----------
% 上一拍已经故障，或者当前触发硬限位，则继续保持故障
fault_latch_now = (travel_fault_latch_z > 0.5) || hard_fault_raw;

% ---------- 3. 软限位方向性限制 ----------
right_soft = (x_mm >= X_max_soft);
left_soft  = (x_mm <= X_min_soft);

v_pos_dir = (v_ref >  V_eps);
v_neg_dir = (v_ref < -V_eps);

right_block = right_soft && v_pos_dir;
left_block  = left_soft  && v_neg_dir;

soft_block = right_block || left_block;

% ---------- 4. 输出安全速度 ----------
if fault_latch_now
    v_ref_safe = 0.0;
elseif soft_block
    v_ref_safe = 0.0;
else
    v_ref_safe = v_ref;
end

travel_fault_latch = double(fault_latch_now);
end

== stateflow chart PMSLM_Close_Loop_MBDL4/FOC_3Close_Loop_Control/Angle_Init ==
  note: 固定电角度，缓慢建立 d 轴电流。
  note: 保持固定电角度，让动子吸附稳定。
  state HOLD_ALIGN
    entry:
    Angle_Init_EN   = 1;
    Init_Done       = 0;
    id_init_ref     = Id_Init_Target;
    Init_State_Num  = 2;
    during:
    Angle_Init_EN = 1;
    Init_Done     = 0;
    id_init_ref   = Id_Init_Target;
  state IDLE
    entry:
    Angle_Init_EN   = 0;
    Init_Done       = 0;
    id_init_ref     = 0;
    Init_State_Num  = 0;
  state RAMP_ID
    entry:
    Angle_Init_EN   = 1;
    Init_Done       = 0;
    id_init_ref     = 0;
    Init_State_Num  = 1;
    during:
    Angle_Init_EN = 1;
    Init_Done     = 0;
    id_init_ref = id_init_ref + Id_Init_Step;
    if (id_init_ref > Id_Init_Target)
    id_init_ref = Id_Init_Target;
    end
  state DONE
    entry:
    Angle_Init_EN   = 0;
    Init_Done       = 1;
    id_init_ref     = 0;
    Init_State_Num  = 3;
    during:
    Angle_Init_EN = 0;
    Init_Done = 1;
    id_init_ref = 0;
    Init_State_Num = 3;
    Theta_Offset_auto = theta_offset_mem;
  HOLD_ALIGN -> IDLE [order 1] : [Init_Reset > 0.5 || travel_fault_latch > 0.5]
  RAMP_ID -> IDLE [order 1] : [Init_Reset > 0.5 || travel_fault_latch > 0.5]
  (default) -> IDLE
  RAMP_ID -> HOLD_ALIGN [order 2] : [after(Ramp_Ticks, tick)]
  IDLE -> RAMP_ID : [Init_Start > 0.5 && Init_Reset < 0.5 && travel_fault_latch < 0.5]
  DONE -> IDLE : [Init_Reset > 0.5 || travel_fault_latch > 0.5]
  HOLD_ALIGN -> DONE [order 2] : [after(Hold_Ticks, tick)]
      | {x_align_mm_latch = x_mm;
      | theta_offset_mem = mod(theta_align_const - 2*pi*x_align_mm_latch/Tau_e_mm, 2*pi);
      | Theta_Offset_auto = theta_offset_mem;}
  data: Init_Start input; Init_Reset input; travel_fault_latch input; Init_Done output; Init_State_Num output; theta_align_const parameter; Tau_e_mm parameter; Id_Init_Target parameter; Ramp_Ticks parameter; Hold_Ticks parameter; Id_Init_Step parameter; id_init_ref output; Angle_Init_EN output; x_mm input; Theta_Offset_auto output; x_align_mm_latch output; theta_offset_mem local
